simulink model "Hybrid_Fuzzy_PI"  (R2020a)
settings: Solver=VariableStepAuto  StartTime=0.0  StopTime=50  FixedStep=0.01  MaxStep=0.1  RelTol=1e-3
values from neighbouring files (symbols this model uses):
  ki_base = 1.2    [DATA_TO_USE.mat]
  kp_base = 0.35    [DATA_TO_USE.mat]
undefined symbols (not defined in the file or in its folder): KENNLINIE_IDENT
libraries: fuzblock x1

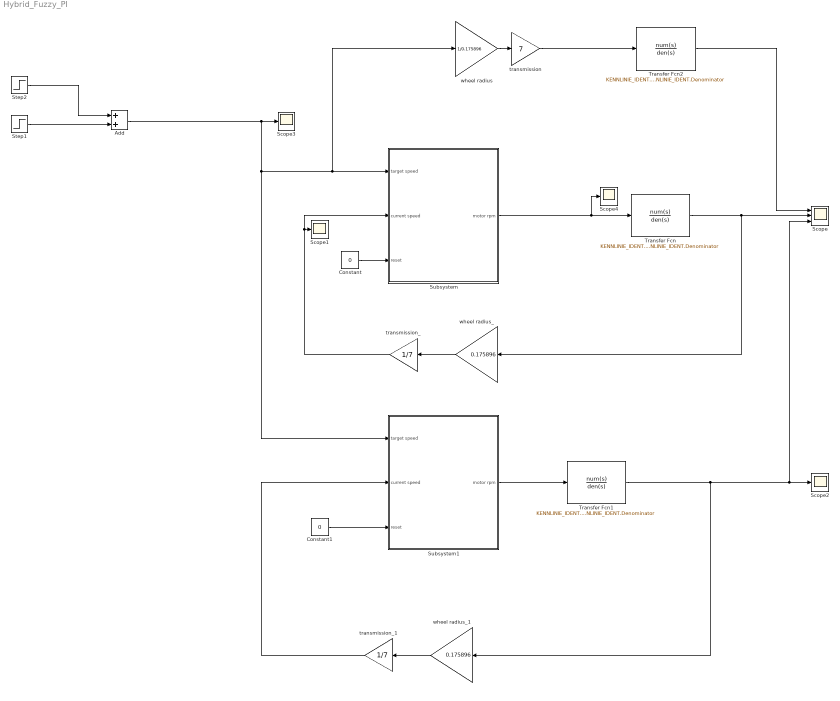
== system Hybrid_Fuzzy_PI ==
  Add : Sum
  Constant : Constant  Value=0
  Constant1 : Constant  Value=0
  Scope : Scope  NumInputPorts=3
  Scope{1..4} (4 alike) : Scope
  Step1 : Step  SampleTime=0
  Step2 : Step  Time=15  After=-0.3  SampleTime=0
  Subsystem : Subsystem
  Subsystem1 : Subsystem
  Transfer Fcn : TransferFcn  Numerator=KENNLINIE_IDENT.Numerator  Denominator=KENNLINIE_IDENT.Denominator
  Transfer Fcn1 : TransferFcn  Numerator=KENNLINIE_IDENT.Numerator  Denominator=KENNLINIE_IDENT.Denominator
  Transfer Fcn2 : TransferFcn  Numerator=KENNLINIE_IDENT.Numerator  Denominator=KENNLINIE_IDENT.Denominator
  transmission : Gain  Gain=7
  transmission_ : Gain  Gain=1/7
  transmission_1 : Gain  Gain=1/7
  wheel radius : Gain  Gain=1/0.175896
  wheel radius_ : Gain  Gain=0.175896
  wheel radius_1 : Gain  Gain=0.175896
  wires:
  Constant/1 -> Subsystem/3("reset ")
  wheel radius_/1 -> transmission_/1
  Transfer Fcn/1 -> wheel radius_/1, Scope/2
  Transfer Fcn1/1 -> wheel radius_1/1, Scope/3, Scope2/1
  Subsystem1/1("motor rpm ") -> Transfer Fcn1/1
  wheel radius_1/1 -> transmission_1/1
  transmission_1/1 -> Subsystem1/2("current speed ")
  Constant1/1 -> Subsystem1/3("reset ")
  Step2/1 -> Add/1
  Step1/1 -> Add/2
  Add/1 -> Scope3/1, Subsystem1/1("target speed "), wheel radius/1, Subsystem/1("target speed ")
  Subsystem/1("motor rpm ") -> Scope4/1, Transfer Fcn/1
  transmission_/1 -> Subsystem/2("current speed "), Scope1/1
  Transfer Fcn2/1 -> Scope/1
  wheel radius/1 -> transmission/1
  transmission/1 -> Transfer Fcn2/1

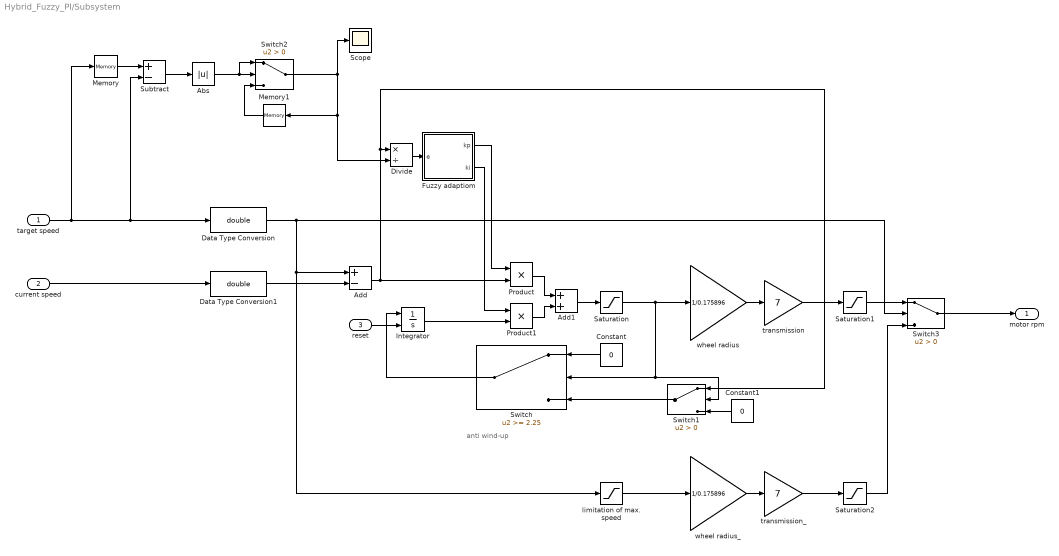
== system Hybrid_Fuzzy_PI/Subsystem ==
  note: anti wind-up
  "target speed " : Inport
  "current speed " : Inport  Port=2
  "reset " : Inport  Port=3
  Abs : Abs
  Add : Sum  Inputs=+-
  Add1 : Sum
  Constant : Constant  Value=0
  Constant1 : Constant  Value=0
  Data Type Conversion : DataTypeConversion  OutDataTypeStr=double
  Data Type Conversion1 : DataTypeConversion  OutDataTypeStr=double
  Divide : Product  Inputs=*/
  "Fuzzy adaptiom " : Subsystem
  Integrator : Integrator  ExternalReset=either
  Memory : Memory  InheritSampleTime=on
  Memory1 : Memory  InheritSampleTime=on
  Product : Product
  Product1 : Product
  Saturation : Saturate  UpperLimit=2.3  LowerLimit=0
  Saturation1 : Saturate  UpperLimit=inf  LowerLimit=0
  Saturation2 : Saturate  UpperLimit=0  LowerLimit=-inf
  Scope : Scope
  Subtract : Sum  Inputs=+-
  Switch : Switch  Threshold=2.25
  Switch1 : Switch  Criteria=u2 > Threshold
  Switch2 : Switch  Criteria=u2 > Threshold
  Switch3 : Switch  Criteria=u2 > Threshold
  limitation of max. speed : Saturate  UpperLimit=0  LowerLimit=-2.3
  transmission : Gain  Gain=7
  transmission_ : Gain  Gain=7
  wheel radius : Gain  Gain=1/0.175896
  wheel radius_ : Gain  Gain=1/0.175896
  "motor rpm " : Outport
  wires:
  "current speed "/1 -> Data Type Conversion1/1
  Saturation1/1 -> Switch3/1
  wheel radius_/1 -> transmission_/1
  Add1/1 -> Saturation/1
  Data Type Conversion/1 -> Switch3/2, Add/1, limitation of max. speed/1
  Switch/1 -> Integrator/1
  "reset "/1 -> Integrator/2
  Data Type Conversion1/1 -> Add/2
  Constant/1 -> Switch/1
  Constant1/1 -> Switch1/3
  Switch3/1 -> "motor rpm "/1
  Product/1 -> Add1/1
  limitation of max. speed/1 -> wheel radius_/1
  Saturation2/1 -> Switch3/3
  transmission/1 -> Saturation1/1
  "target speed "/1 -> Memory/1, Subtract/2, Data Type Conversion/1
  transmission_/1 -> Saturation2/1
  Product1/1 -> Add1/2
  Saturation/1 -> Switch/2, Switch1/2, wheel radius/1
  Switch1/1 -> Switch/3
  wheel radius/1 -> transmission/1
  Add/1 -> Divide/1, Switch1/1, Product/2
  Integrator/1 -> Product1/2
  "Fuzzy adaptiom "/1(kp) -> Product/1
  "Fuzzy adaptiom "/2(ki) -> Product1/1
  Memory/1 -> Subtract/1
  Subtract/1 -> Abs/1
  Abs/1 -> Switch2/1, Switch2/2
  Switch2/1 -> Scope/1, Divide/2, Memory1/1
  Memory1/1 -> Switch2/3
  Divide/1 -> "Fuzzy adaptiom "/1(e)

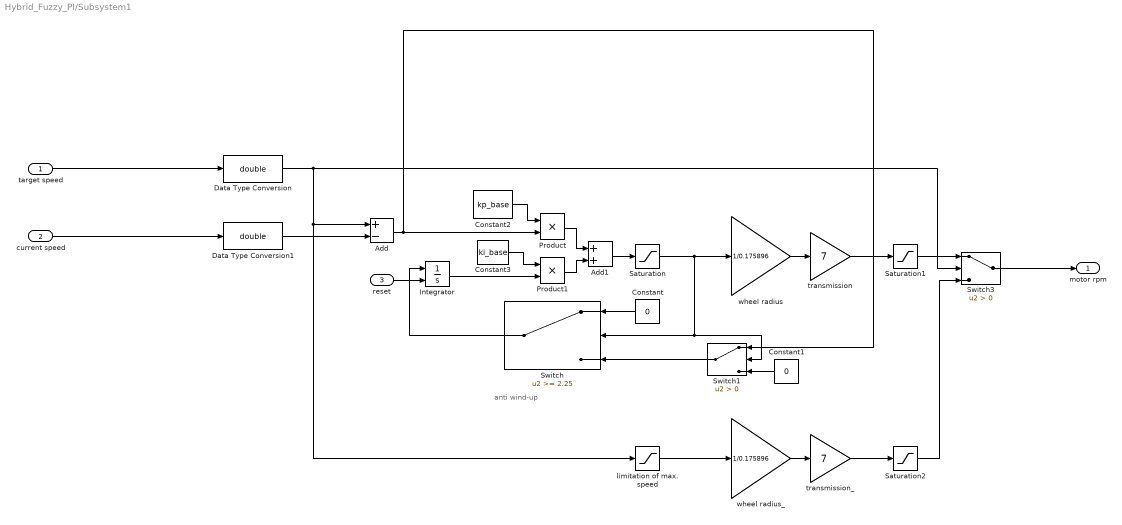
== system Hybrid_Fuzzy_PI/Subsystem1 ==
  note: anti wind-up
  "target speed " : Inport
  "current speed " : Inport  Port=2
  "reset " : Inport  Port=3
  Add : Sum  Inputs=+-
  Add1 : Sum
  Constant : Constant  Value=0
  Constant1 : Constant  Value=0
  Constant2 : Constant  Value=kp_base
  Constant3 : Constant  Value=ki_base
  Data Type Conversion : DataTypeConversion  OutDataTypeStr=double
  Data Type Conversion1 : DataTypeConversion  OutDataTypeStr=double
  Integrator : Integrator  ExternalReset=either
  Product : Product
  Product1 : Product
  Saturation : Saturate  UpperLimit=2.3  LowerLimit=0
  Saturation1 : Saturate  UpperLimit=inf  LowerLimit=0
  Saturation2 : Saturate  UpperLimit=0  LowerLimit=-inf
  Switch : Switch  Threshold=2.25
  Switch1 : Switch  Criteria=u2 > Threshold
  Switch3 : Switch  Criteria=u2 > Threshold
  limitation of max. speed : Saturate  UpperLimit=0  LowerLimit=-2.3
  transmission : Gain  Gain=7
  transmission_ : Gain  Gain=7
  wheel radius : Gain  Gain=1/0.175896
  wheel radius_ : Gain  Gain=1/0.175896
  "motor rpm " : Outport
  wires:
  "current speed "/1 -> Data Type Conversion1/1
  Saturation1/1 -> Switch3/1
  wheel radius_/1 -> transmission_/1
  Add1/1 -> Saturation/1
  Data Type Conversion/1 -> Switch3/2, Add/1, limitation of max. speed/1
  Switch/1 -> Integrator/1
  "reset "/1 -> Integrator/2
  Data Type Conversion1/1 -> Add/2
  Constant/1 -> Switch/1
  Constant1/1 -> Switch1/3
  Switch3/1 -> "motor rpm "/1
  Product/1 -> Add1/1
  limitation of max. speed/1 -> wheel radius_/1
  Saturation2/1 -> Switch3/3
  transmission/1 -> Saturation1/1
  "target speed "/1 -> Data Type Conversion/1
  transmission_/1 -> Saturation2/1
  Product1/1 -> Add1/2
  Saturation/1 -> Switch/2, Switch1/2, wheel radius/1
  Switch1/1 -> Switch/3
  wheel radius/1 -> transmission/1
  Add/1 -> Switch1/1, Product/2
  Integrator/1 -> Product1/2
  Constant2/1 -> Product/1
  Constant3/1 -> Product1/1

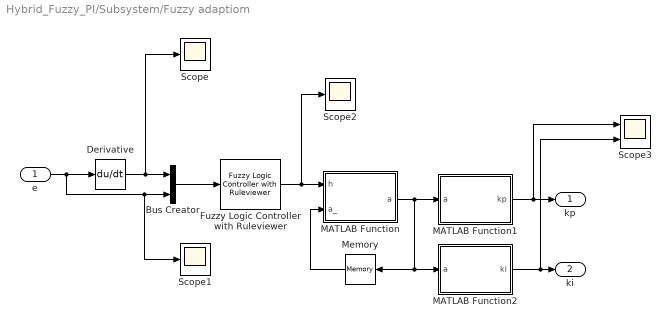
== system Hybrid_Fuzzy_PI/Subsystem/Fuzzy adaptiom  ==
  e : Inport
  Bus Creator : BusCreator  Inputs=2
  Derivative : Derivative
  Fuzzy Logic Controller with Ruleviewer : fuzblock/Fuzzy Logic  Controller  with Ruleviewer  fismatrix=Fuzzy2  Ts=2
  MATLAB Function : MATLAB Function  TreatAsAtomicUnit=on
  MATLAB Function1 : MATLAB Function  TreatAsAtomicUnit=on
  MATLAB Function2 : MATLAB Function  TreatAsAtomicUnit=on
  Memory : Memory  InitialCondition=0.5
  Scope : Scope
  Scope1 : Scope
  Scope2 : Scope
  Scope3 : Scope  NumInputPorts=2
  kp : Outport
  ki : Outport  Port=2
  wires:
  Bus Creator/1 -> Fuzzy Logic Controller with Ruleviewer/1
  Fuzzy Logic Controller with Ruleviewer/1 -> Scope2/1, MATLAB Function/1(h)
  MATLAB Function/1(a) -> MATLAB Function1/1(a), MATLAB Function2/1(a), Memory/1
  Derivative/1 -> Scope/1, Bus Creator/1
  Memory/1 -> MATLAB Function/2(a_)
  e/1 -> Scope1/1, Bus Creator/2, Derivative/1
  MATLAB Function1/1(kp) -> Scope3/1, kp/1
  MATLAB Function2/1(ki) -> Scope3/2, ki/1

== matlab function Hybrid_Fuzzy_PI/Subsystem/Fuzzy adaptiom /MATLAB Function ==
function a = fcn(h, a_)
    y=0.1;
    if a_ > 0.5
        a = a_ + y * h * (1 - a_);  
    else
        a = a_ + y * h * a_; 
    end

== matlab function Hybrid_Fuzzy_PI/Subsystem/Fuzzy adaptiom /MATLAB Function2 ==
function ki = fcn(a)
ki_base =1.2 ;%defined by PID-Tuner
ki = a*ki_base*(1+a);

== matlab function Hybrid_Fuzzy_PI/Subsystem/Fuzzy adaptiom /MATLAB Function1 ==
function kp = fcn(a)
ku = 0.35;%defined by PID-Tuner
kp = ku*a;
